simulink library "DQN_Lib"  (R2023b)
settings: Solver=VariableStepAuto  StartTime=0.0  StopTime=10.0  RelTol=1e-3
undefined symbols (not defined in the file): ACDC3, HRM, La, N, R, Ra, sps_AC, SYS, Ts, Ts_dqn, Ts_Power, w, Ws
libraries: DQN_Lib_bak x7
(part 2 of 3)

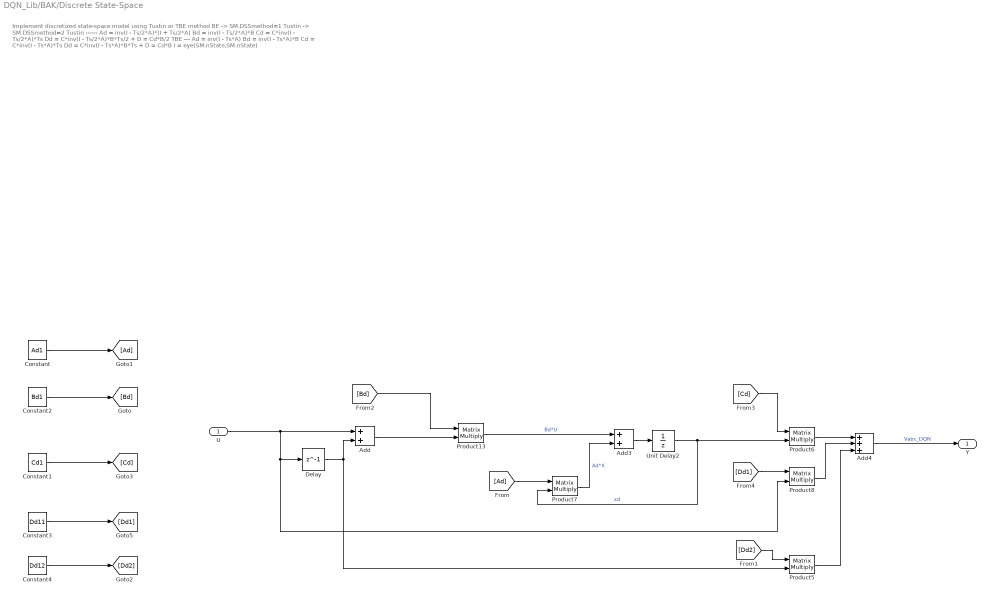
== system DQN_Lib/BAK/Discrete State-Space ==
  note: Implement discretized state-space model using Tustin or TBE method
      |
      | BE      -> SM.DSSmethod=1
      | Tustin  -> SM.DSSmethod=2
      |
      |
      | Tustin
      | ------
      | Ad = inv(I - Ts/2*A)*(I + Ts/2*A)
      | Bd = inv(I - Ts/2*A)*B
      | Cd = C*inv(I - Ts/2*A)*Ts
      | Dd = C*inv(I - Ts/2*A)*B*Ts/2  + D  =  Cd*B/2
      |
      | TBE
      | ---
      | Ad = inv(I - Ts*A)
      | Bd = inv(I - Ts*A)*B
      | Cd = C*inv(I - Ts*A)*Ts
      | Dd = C*inv(I - Ts*A)*B*Ts  + D  =  Cd*B
      |
      | I = eye(SM.nState,SM.nState)
  U : Inport
  Add : Sum
  Add3 : Sum
  Add4 : Sum  Inputs=+++
  Constant : Constant  Value=Ad1
  Constant1 : Constant  Value=Cd1
  Constant2 : Constant  Value=Bd1
  Constant3 : Constant  Value=Dd11
  Constant4 : Constant  Value=Dd12
  Delay : Delay  DelayLength=1  SampleTime=dt
  Product{5..8,13} (5 alike) : Product  Multiplication=Matrix(*)  SaturateOnIntegerOverflow=on  OutDataTypeStr=Inherit: Same as first input
  Unit Delay2 : UnitDelay  InitialCondition=InitVec  SampleTime=dt  HasFrameUpgradeWarning=on
  Y : Outport
  wires:
  Add3/1 -> Unit Delay2/1
  Delay/1 -> Add/2, Product5/2
  [Cd] -> Product6/1
  Unit Delay2/1 -> Product6/2, Product7/2  "xd"
  Product6/1 -> Add4/1
  Add/1 -> Product13/2
  Product7/1 -> Add3/2  "Ad*X"
  Product13/1 -> Add3/1  "Bd*U"
  [Bd] -> Product13/1
  U/1 -> Delay/1, Product8/2, Add/1
  [Dd1] -> Product8/1
  [Ad] -> Product7/1
  Product8/1 -> Add4/2
  Product5/1 -> Add4/3
  [Dd2] -> Product5/1
  Add4/1 -> Y/1  "Vabc_DQN"
  Constant/1 -> [Ad]
  Constant2/1 -> [Bd]
  Constant1/1 -> [Cd]
  Constant3/1 -> [Dd1]
  Constant4/1 -> [Dd2]

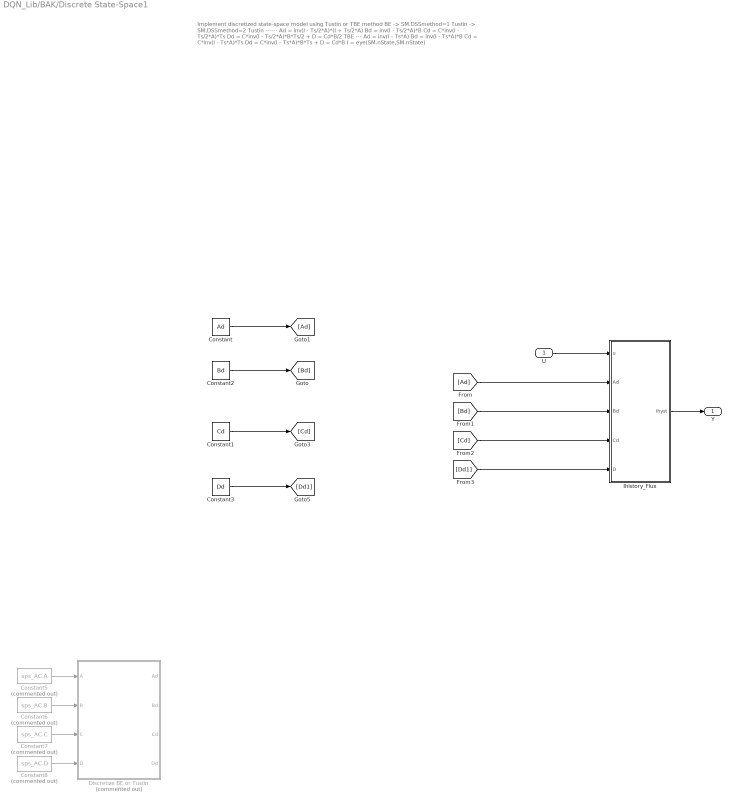
== system DQN_Lib/BAK/Discrete State-Space1 ==
  note: Implement discretized state-space model using Tustin or TBE method
      |
      | BE      -> SM.DSSmethod=1
      | Tustin  -> SM.DSSmethod=2
      |
      |
      | Tustin
      | ------
      | Ad = inv(I - Ts/2*A)*(I + Ts/2*A)
      | Bd = inv(I - Ts/2*A)*B
      | Cd = C*inv(I - Ts/2*A)*Ts
      | Dd = C*inv(I - Ts/2*A)*B*Ts/2  + D  =  Cd*B/2
      |
      | TBE
      | ---
      | Ad = inv(I - Ts*A)
      | Bd = inv(I - Ts*A)*B
      | Cd = C*inv(I - Ts*A)*Ts
      | Dd = C*inv(I - Ts*A)*B*Ts  + D  =  Cd*B
      |
      | I = eye(SM.nState,SM.nState)
  U : Inport
  Constant : Constant  Value=Ad
  Constant1 : Constant  Value=Cd
  Constant2 : Constant  Value=Bd
  Constant3 : Constant  Value=Dd
  Constant5 : Constant  Commented=on  Value=sps_AC.A
  Constant6 : Constant  Commented=on  Value=sps_AC.B
  Constant7 : Constant  Commented=on  Value=sps_AC.C
  Constant8 : Constant  Commented=on  Value=sps_AC.D
  Discretize BE or Tustin : Subsystem  Commented=on  AncestorBlock="DQN_Machines/DQN_Mac_V1/Discretize  BE or Tustin"
  Ihistory_Flux : Subsystem  AncestorBlock=DQN_Machines/DQN_Mac_V1/Ihistory_Flux
  Y : Outport
  wires:
  Constant/1 -> [Ad]
  Constant2/1 -> [Bd]
  Constant1/1 -> [Cd]
  Constant3/1 -> [Dd1]
  Constant7/1 -> Discretize BE or Tustin/3(C)
  Constant6/1 -> Discretize BE or Tustin/2(B)
  Constant8/1 -> Discretize BE or Tustin/4(D)
  Constant5/1 -> Discretize BE or Tustin/1(A)
  U/1 -> Ihistory_Flux/1(u)
  Ihistory_Flux/1(Ihyst) -> Y/1
  [Ad] -> Ihistory_Flux/2(Ad)
  [Bd] -> Ihistory_Flux/3(Bd)
  [Cd] -> Ihistory_Flux/4(Cd)
  [Dd1] -> Ihistory_Flux/5(D)

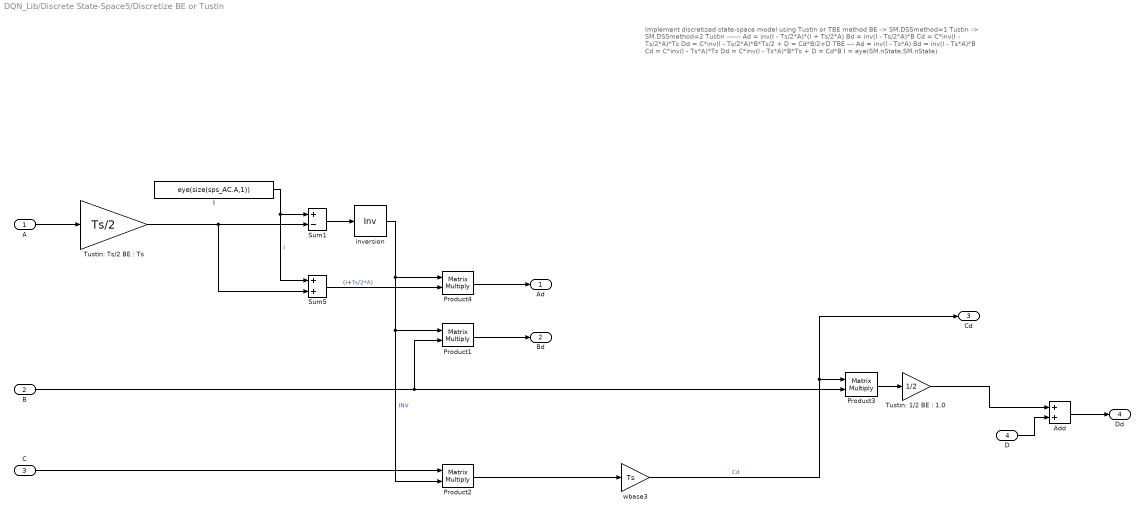
== system DQN_Lib/Discrete State-Space5/Discretize BE or Tustin ==
  note: Implement discretized state-space model using Tustin or TBE method
      |
      | BE      -> SM.DSSmethod=1
      | Tustin  -> SM.DSSmethod=2
      |
      |
      | Tustin
      | ------
      | Ad = inv(I - Ts/2*A)*(I + Ts/2*A)
      | Bd = inv(I - Ts/2*A)*B
      | Cd = C*inv(I - Ts/2*A)*Ts
      | Dd = C*inv(I - Ts/2*A)*B*Ts/2  + D  =  Cd*B/2+D
      |
      | TBE
      | ---
      | Ad = inv(I - Ts*A)
      | Bd = inv(I - Ts*A)*B
      | Cd = C*inv(I - Ts*A)*Ts
      | Dd = C*inv(I - Ts*A)*B*Ts  + D  =  Cd*B
      |
      | I = eye(SM.nState,SM.nState)
  A : Inport
  B : Inport  Port=2
  C : Inport  Port=3
  D : Inport  Port=4
  Add : Sum
  I : Constant  Value=eye(size(sps_AC.A,1))
  Product{1..4} (4 alike) : Product  Multiplication=Matrix(*)  SaturateOnIntegerOverflow=on  OutDataTypeStr=Inherit: Same as first input
  Sum1 : Sum  Inputs=+-  SaturateOnIntegerOverflow=on
  Sum5 : Sum  SaturateOnIntegerOverflow=on
  "Tustin: 1/2 BE : 1.0" : Gain  Gain=1/2  SaturateOnIntegerOverflow=on  OutDataTypeStr=Inherit: Same as input  ParamDataTypeStr=Inherit: Same as input
  "Tustin: Ts/2 BE : Ts" : Gain  Gain=Ts/2  SaturateOnIntegerOverflow=on  OutDataTypeStr=Inherit: Same as input  ParamDataTypeStr=Inherit: Same as input
  inversion : Product  Inputs=/  Multiplication=Matrix(*)  RndMeth=Zero
  wbase3 : Gain  Gain=Ts  SaturateOnIntegerOverflow=on  OutDataTypeStr=Inherit: Same as input  ParamDataTypeStr=Inherit: Same as input
  Ad : Outport  VectorParamsAs1DForOutWhenUnconnected=off
  Bd : Outport  Port=2  VectorParamsAs1DForOutWhenUnconnected=off
  Cd : Outport  Port=3  VectorParamsAs1DForOutWhenUnconnected=off
  Dd : Outport  Port=4  VectorParamsAs1DForOutWhenUnconnected=off
  wires:
  D/1 -> Add/2
  Add/1 -> Dd/1
  "Tustin: Ts/2 BE : Ts"/1 -> Sum1/2, Sum5/2
  Product4/1 -> Ad/1
  A/1 -> "Tustin: Ts/2 BE : Ts"/1
  I/1 -> Sum5/1, Sum1/1  "I"
  Sum1/1 -> inversion/1
  inversion/1 -> Product2/2, Product1/1, Product4/1  "INV"
  Sum5/1 -> Product4/2  "(I+Ts/2*A)"
  Product1/1 -> Bd/1
  B/1 -> Product1/2, Product3/2
  C/1 -> Product2/1
  Product3/1 -> "Tustin: 1/2 BE : 1.0"/1
  "Tustin: 1/2 BE : 1.0"/1 -> Add/1
  Product2/1 -> wbase3/1
  wbase3/1 -> Cd/1, Product3/1  "Cd"

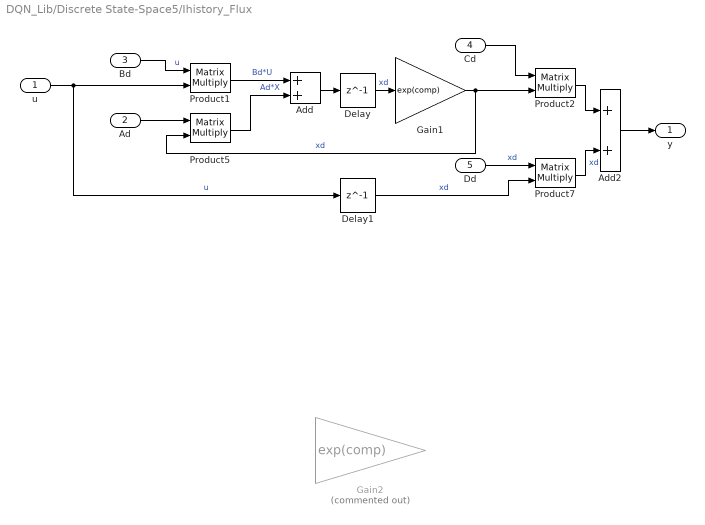
== system DQN_Lib/Discrete State-Space5/Ihistory_Flux ==
  u : Inport
  Ad : Inport  Port=2
  Bd : Inport  Port=3
  Cd : Inport  Port=4
  Dd : Inport  Port=5
  Add : Sum
  Add2 : Sum
  Delay : Delay  DelayLength=1  InitialCondition=InitVec  SampleTime=dt
  Delay1 : Delay  DelayLength=1  InitialCondition=0  SampleTime=dt
  Gain1 : Gain  Gain=exp(comp)
  Gain2 : Gain  Commented=on  Gain=exp(comp)
  Product{1..2,5,7} (4 alike) : Product  Multiplication=Matrix(*)  SaturateOnIntegerOverflow=on  OutDataTypeStr=Inherit: Same as first input
  y : Outport  VectorParamsAs1DForOutWhenUnconnected=off
  wires:
  Dd/1 -> Product7/1  "xd"
  Product7/1 -> Add2/2  "xd"
  Cd/1 -> Product2/1
  Ad/1 -> Product5/1
  Product5/1 -> Add/2  "Ad*X"
  Delay/1 -> Gain1/1  "xd"
  Add/1 -> Delay/1
  Product1/1 -> Add/1  "Bd*U"
  Product2/1 -> Add2/1
  u/1 -> Delay1/1, Product1/2  "u"
  Bd/1 -> Product1/1  "u"
  Add2/1 -> y/1
  Gain1/1 -> Product2/2, Product5/2  "xd"
  Delay1/1 -> Product7/2  "xd"

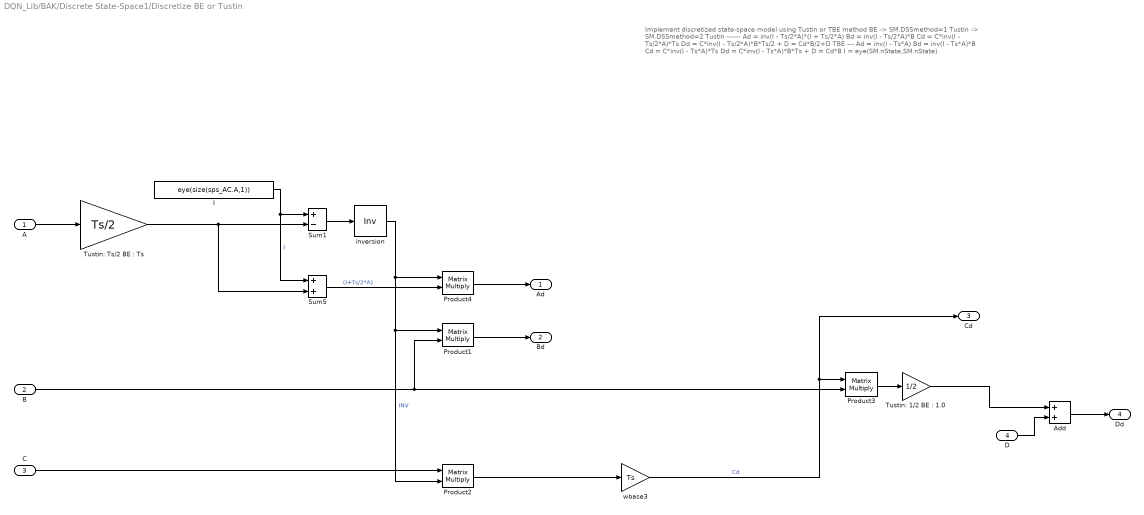
== system DQN_Lib/BAK/Discrete State-Space1/Discretize BE or Tustin ==
  note: Implement discretized state-space model using Tustin or TBE method
      |
      | BE      -> SM.DSSmethod=1
      | Tustin  -> SM.DSSmethod=2
      |
      |
      | Tustin
      | ------
      | Ad = inv(I - Ts/2*A)*(I + Ts/2*A)
      | Bd = inv(I - Ts/2*A)*B
      | Cd = C*inv(I - Ts/2*A)*Ts
      | Dd = C*inv(I - Ts/2*A)*B*Ts/2  + D  =  Cd*B/2+D
      |
      | TBE
      | ---
      | Ad = inv(I - Ts*A)
      | Bd = inv(I - Ts*A)*B
      | Cd = C*inv(I - Ts*A)*Ts
      | Dd = C*inv(I - Ts*A)*B*Ts  + D  =  Cd*B
      |
      | I = eye(SM.nState,SM.nState)
  A : Inport
  B : Inport  Port=2
  C : Inport  Port=3
  D : Inport  Port=4
  Add : Sum
  I : Constant  Value=eye(size(sps_AC.A,1))
  Product{1..4} (4 alike) : Product  Multiplication=Matrix(*)  SaturateOnIntegerOverflow=on  OutDataTypeStr=Inherit: Same as first input
  Sum1 : Sum  Inputs=+-  SaturateOnIntegerOverflow=on
  Sum5 : Sum  SaturateOnIntegerOverflow=on
  "Tustin: 1/2 BE : 1.0" : Gain  Gain=1/2  SaturateOnIntegerOverflow=on  OutDataTypeStr=Inherit: Same as input  ParamDataTypeStr=Inherit: Same as input
  "Tustin: Ts/2 BE : Ts" : Gain  Gain=Ts/2  SaturateOnIntegerOverflow=on  OutDataTypeStr=Inherit: Same as input  ParamDataTypeStr=Inherit: Same as input
  inversion : Product  Inputs=/  Multiplication=Matrix(*)  RndMeth=Zero
  wbase3 : Gain  Gain=Ts  SaturateOnIntegerOverflow=on  OutDataTypeStr=Inherit: Same as input  ParamDataTypeStr=Inherit: Same as input
  Ad : Outport  VectorParamsAs1DForOutWhenUnconnected=off
  Bd : Outport  Port=2  VectorParamsAs1DForOutWhenUnconnected=off
  Cd : Outport  Port=3  VectorParamsAs1DForOutWhenUnconnected=off
  Dd : Outport  Port=4  VectorParamsAs1DForOutWhenUnconnected=off
  wires:
  wbase3/1 -> Product3/1, Cd/1  "Cd"
  Product2/1 -> wbase3/1
  "Tustin: 1/2 BE : 1.0"/1 -> Add/1
  Product3/1 -> "Tustin: 1/2 BE : 1.0"/1
  C/1 -> Product2/1
  B/1 -> Product3/2, Product1/2
  Product1/1 -> Bd/1
  Sum5/1 -> Product4/2  "(I+Ts/2*A)"
  inversion/1 -> Product4/1, Product1/1, Product2/2  "INV"
  Sum1/1 -> inversion/1
  I/1 -> Sum1/1, Sum5/1  "I"
  A/1 -> "Tustin: Ts/2 BE : Ts"/1
  Product4/1 -> Ad/1
  "Tustin: Ts/2 BE : Ts"/1 -> Sum5/2, Sum1/2
  Add/1 -> Dd/1
  D/1 -> Add/2

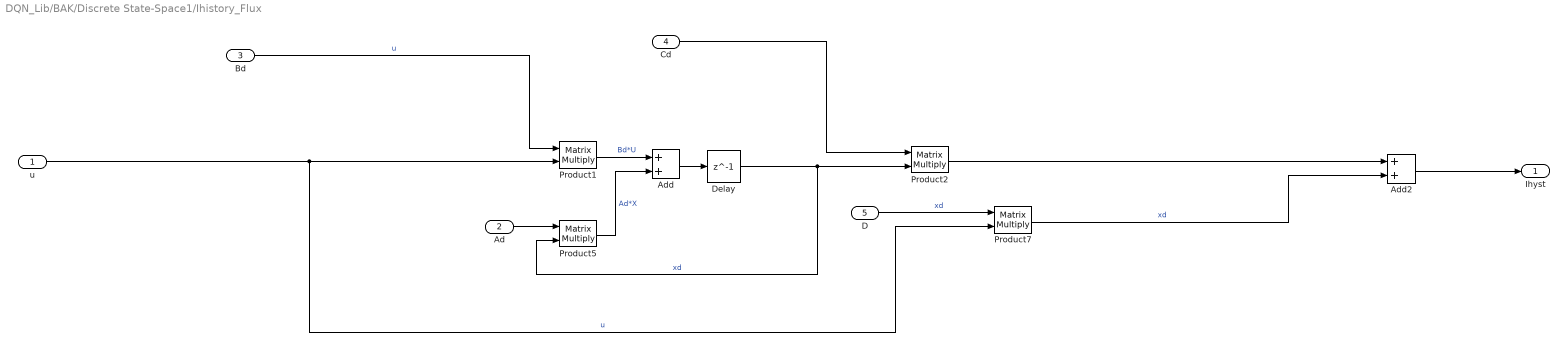
== system DQN_Lib/BAK/Discrete State-Space1/Ihistory_Flux ==
  u : Inport
  Ad : Inport  Port=2
  Bd : Inport  Port=3
  Cd : Inport  Port=4
  D : Inport  Port=5
  Add : Sum
  Add2 : Sum
  Delay : Delay  DelayLength=1  InitialCondition=InitVec  SampleTime=dt
  Product{1..2,5,7} (4 alike) : Product  Multiplication=Matrix(*)  SaturateOnIntegerOverflow=on  OutDataTypeStr=Inherit: Same as first input
  Ihyst : Outport  VectorParamsAs1DForOutWhenUnconnected=off
  wires:
  Add2/1 -> Ihyst/1
  Bd/1 -> Product1/1  "u"
  u/1 -> Product7/2, Product1/2  "u"
  Product2/1 -> Add2/1
  Product1/1 -> Add/1  "Bd*U"
  Add/1 -> Delay/1
  Delay/1 -> Product2/2, Product5/2  "xd"
  Product5/1 -> Add/2  "Ad*X"
  Ad/1 -> Product5/1
  Cd/1 -> Product2/1
  Product7/1 -> Add2/2  "xd"
  D/1 -> Product7/1  "xd"

== matlab function DQN_Lib/MATLAB Function2 ==
  data: Ydcpnz_c output; X_DQN input; N parameter
function Ydcpnz_c  = fDQN012C(X_DQN, N)
        
            if(size(X_DQN,2) < 1)
                error('Wrong size!');
            end
            
            % N = size(X_DQN,1);
            % 
            % if(size(X_DQN,1) == 6 && size(X_DQN,2) == 1)
            %     N = 1;
            %     X_DQN = X_DQN';
            % end
        
            Ydcpnz_c = complex(zeros(3,N+1));
        
            for i = 1 : N+1
             
                if(i>1)
                    Ydcpnz_c(1,i) = (X_DQN(i,1)) + 1i*X_DQN(i,4);
                    Ydcpnz_c(2,i) = (-X_DQN(i,2)) + 1i*X_DQN(i,5);
                    Ydcpnz_c(3,i) = (X_DQN(i,3)) + 1i*X_DQN(i,6);
                else
        
                    Ydcpnz_c(1,i) = 0.5*(X_DQN(i,4) - 1i*X_DQN(i,1));
                    Ydcpnz_c(2,i) = 0.5*(X_DQN(i,5) + 1i*X_DQN(i,2));
                    Ydcpnz_c(3,i) =     (X_DQN(i,6) + 1i*X_DQN(i,3));
                end
            
            end
        
        
        end

== matlab function DQN_Lib/Subsystem1/DQN Mux ==
  data: u input; y output; N parameter
function y = MUX_vec(u, N)

    y = zeros((N+1)*6,1);

    for i = 1 : (N+1)*6


        if(i <= 1*(N+1)) %dp
            y(i) = u(mod(i+N,N+1)*6+1);
        elseif(i > 1*(N+1) && i <= 2*(N+1))
            y(i) = u(mod(i+N,N+1)*6+2);
        elseif(i > 2*(N+1) && i <= 3*(N+1))
            y(i) = u(mod(i+N,N+1)*6+3);
        elseif(i > 3*(N+1) && i <= 4*(N+1))
            y(i) = u(mod(i+N,N+1)*6+4);
        elseif(i > 4*(N+1) && i <= 5*(N+1))
            y(i) = u(mod(i+N,N+1)*6+5);
        elseif(i > 5*(N+1) && i <= 6*(N+1))
            y(i) = u(mod(i+N,N+1)*6+6);
        end
    end
    
end

== matlab function DQN_Lib/ABC2PNZ ==
  data: Xabc input; Ypnz output
function Ypnz  = ABC2PNZ(Xabc)
    persistent Sas;

    if(isempty(Sas)) 
        a = -0.5+0.866i;
        a2 = -0.5-0.866i;
        Sas = [1,a,a2;1,a2,a;1,1,1]/3;
    end
    
    Ypnz = Sas*Xabc/Sas;

end

== matlab function DQN_Lib/Int_DQN_fdbk/Int_d_2N_2 ==
  settings: updateMethod=DISCRETE
  data: Zdp output; Xdp input; Xdn input; Xdz input; Xqp input; Xqn input; Xqz input; Zdn output; N parameter; dt parameter; w parameter; Zdz output; Zqp output; Zqn output; Zqz output; R parameter; iL parameter; SW parameter
function [Zdp,Zdn,Zdz,Zqp,Zqn,Zqz]  = IntDQN(Xdp, Xdn, Xdz, Xqp, Xqn, Xqz, N, dt, w, R, iL, SW)

    persistent Zdc_old;    
    persistent Xdc_old;   
    persistent Zdp_old;    
    persistent Zqp_old;    
    persistent Zdn_old;    
    persistent Zqn_old;    
    persistent Zdz_old;    
    persistent Zqz_old;  
    persistent Krl1;
    persistent Krl2;
       
    persistent dt2;
    persistent range;
       
    Xdc = zeros(6,1);
    Zdc = zeros(6,1);
    
    Xdc(1) = Xdp(1);
    Xdc(2) = Xdn(1);
    Xdc(3) = Xdz(1);
    Xdc(4) = Xqp(1);
    Xdc(5) = Xqn(1);
    Xdc(6) = Xqz(1);

    Xdp = [Xdp(2:end); zeros(N-numel(Xdp)+1,1)];
    Xqp = [Xqp(2:end); zeros(N-numel(Xqp)+1,1)];
    Xdn = [Xdn(2:end); zeros(N-numel(Xdn)+1,1)];
    Xqn = [Xqn(2:end); zeros(N-numel(Xqn)+1,1)];
    Xdz = [Xdz(2:end); zeros(N-numel(Xdz)+1,1)];
    Xqz = [Xqz(2:end); zeros(N-numel(Xqz)+1,1)];
       
    Zdp = zeros(N+1,1);
    Zdn = zeros(N+1,1);
    Zqp = zeros(N+1,1);
    Zqn = zeros(N+1,1);
    Zdz = zeros(N+1,1);
    Zqz = zeros(N+1,1);
       
    if(isempty(Zdp_old)) 
        Zdc_old  = zeros(6,1); %Zdc_old  = InitInt';
        Xdc_old  = zeros(6,1);
        
        Zdp_old  = zeros(N,1);% Zdp_old(1) = InitInt(1);
        Zdn_old  = zeros(N,1);% Zdn_old(1) = InitInt(2);
        Zdz_old  = zeros(N,1);% Zdz_old(1) = InitInt(3);
        Zqp_old  = zeros(N,1);% Zqp_old(1) = InitInt(4);
        Zqn_old  = zeros(N,1);% Zqn_old(1) = InitInt(5);
        Zqz_old  = zeros(N,1);% Zqz_old(1) = InitInt(6);
        
        dt2 = dt/2;  
        range = N; 
        
        if(SW)
            Krl1 = (iL/(1+dt2*R*iL));
            Krl2 = (1-dt2*R*iL)/(1+dt2*R*iL);
        else
            Krl1 = 1;
            Krl2 = 1;
        end
        
    end

    
    
    %Zdc(:) = dt2*(Xdc(:)+Xdc_old(:))+Zdc_old(:);
    Zdc(:) = Krl1*dt2*(Xdc(:)+Xdc_old(:))+Krl2*Zdc_old(:);
    
    
    Zdc_old = Zdc;
    Xdc_old = Xdc;
    
    if(N>0)
              
        for i = 1 : range

            wn =  i * w;
            wndt2 = wn*dt2;
            A = 2*dt2/(1+wndt2^2);
            B = (1-wndt2^2)/(1+wndt2^2);

            %%% NEG %%%
            Zdp(i) = Krl1*A*(Xdp(i)+wndt2*Xqp(i))+Krl2*(B*Zdp_old(i)+A*wn*Zqp_old(i));
            Zqp(i) = Krl1*A*(Xqp(i)-wndt2*Xdp(i))+Krl2*(B*Zqp_old(i)-A*wn*Zdp_old(i));

            Zdp_old(i) = Zdp(i);
            Zqp_old(i) = Zqp(i); 


            %%% NEG %%%
            Zdn(i) = Krl1*A*(Xdn(i)-wndt2*Xqn(i))+Krl2*(B*Zdn_old(i)-A*wn*Zqn_old(i));
            Zqn(i) = Krl1*A*(Xqn(i)+wndt2*Xdn(i))+Krl2*(B*Zqn_old(i)+A*wn*Zdn_old(i));

            Zdn_old(i) = Zdn(i);
            Zqn_old(i) = Zqn(i); 

            %%% ZERO %%%
            Zdz(i) = Krl1*A*(Xdz(i)+wndt2*Xqz(i))+Krl2*(B*Zdz_old(i)+A*wn*Zqz_old(i));
            Zqz(i) = Krl1*A*(Xqz(i)-wndt2*Xdz(i))+Krl2*(B*Zqz_old(i)-A*wn*Zdz_old(i));

            Zdz_old(i) = Zdz(i);
            Zqz_old(i) = Zqz(i); 
        end

        Zdp(2:end) = Zdp(1:end-1);
        Zdn(2:end) = Zdn(1:end-1);
        Zdz(2:end) = Zdz(1:end-1);
        Zqp(2:end) = Zqp(1:end-1);
        Zqn(2:end) = Zqn(1:end-1);
        Zqz(2:end) = Zqz(1:end-1);


    end
    
    Zdp(1)     = Zdc(1);
    Zdn(1)     = Zdc(2);
    Zdz(1)     = Zdc(3);
    Zqp(1)     = Zdc(4);
    Zqn(1)     = Zdc(5);
    Zqz(1)     = Zdc(6);
end

== matlab function DQN_Lib/MATLAB Function4 ==
  data: Xdcpnz_c input; Y_DQN output
function Y_DQN  = f012C2DQN(Xdcpnz_c)

    if(size(Xdcpnz_c,2) < 2)
        error('Wrong size!');
    end
    
    N = size(Xdcpnz_c,2)-1;
    Y_DQN = zeros(N+1,6);

    Y_DQN(1,4) =  2*real(Xdcpnz_c(1,1));
    Y_DQN(1,5) =  2*real(Xdcpnz_c(2,1));
    Y_DQN(1,6) =  real(Xdcpnz_c(3,1));

    Y_DQN(1,1) =  -2*imag(Xdcpnz_c(1,1));
    Y_DQN(1,2) =  2*imag(Xdcpnz_c(2,1));
    Y_DQN(1,3) =  imag(Xdcpnz_c(3,1));
    
    for i = 2 : N + 1
    
        Y_DQN(i,1) =  real(Xdcpnz_c(1,i));
        Y_DQN(i,2) = -real(Xdcpnz_c(2,i));
        Y_DQN(i,3) =  real(Xdcpnz_c(3,i));

        Y_DQN(i,4) =  imag(Xdcpnz_c(1,i));
        Y_DQN(i,5) =  imag(Xdcpnz_c(2,i));
        Y_DQN(i,6) =  imag(Xdcpnz_c(3,i));
    
    end


end

== matlab function DQN_Lib/Mult_DQNc_Mat ==
  data: Xdcpnz_c input; Ydcpnz_c input; N parameter; HrmDbl parameter; Zdcpnz_c output
function Zdcpnz_c    = fMultDQNc(Xdcpnz_c, Ydcpnz_c, N, HrmDbl)
    Zdcpnz_c = complex(zeros(3,2*N+1));

    persistent T132;
    persistent T213;
    persistent T231;
    persistent T321;
    persistent T312;
    persistent Sas;
    persistent Ssa;

    if(isempty(T132)) 
        T132 = [1 0 0; 0 0 1; 0 1 0];
        T213 = [0 1 0; 1 0 0; 0 0 1];
        T231 = [0 1 0; 0 0 1; 1 0 0];
        T321 = [0 0 1; 0 1 0; 1 0 0];
        T312 = [0 0 1; 1 0 0; 0 1 0];

        a = -0.5+0.866i;
        a2 = -0.5-0.866i;
        Sas = [1,a,a2;1,a2,a;1,1,1]/3;
        Ssa = eye(3)/(Sas);
    end

%%%%%%%%%%%%%%%%%%%%%%%%%%%%%%

    Zdcpnz_c(:,1) = Sas*(Ssa*Xdcpnz_c(:,1).*Ssa*Ydcpnz_c(:,1));

    sX = size(Xdcpnz_c,2);
    Xdcpnz_c = [Xdcpnz_c zeros(3,N+1-sX)];

    sY = size(Ydcpnz_c,2);
    Ydcpnz_c = [Ydcpnz_c zeros(3,N+1-sY)];

       
    for h = 1 : 2*N
        if(h<=N)

            Zdcpnz_c(3,1) = Zdcpnz_c(3,1) + 0.5*real(Xdcpnz_c(:,h+1)'*Ydcpnz_c(:,h+1));


            Zdcpnz_c(3,2*h+1) = Zdcpnz_c(3,2*h+1) + 0.5*Xdcpnz_c(1,h+1)*Ydcpnz_c(2,h+1)*exp(-1i*pi/2);

            Zdcpnz_c(1:2,1) = Zdcpnz_c(1:2,1) + 0.25*abs(Xdcpnz_c(1,h+1))*abs(Ydcpnz_c(2,h+1))*[1;1].*exp(1i*((-angle(Xdcpnz_c(1,h+1))+angle(Ydcpnz_c(2,h+1)))*[1;-1]));
            Zdcpnz_c(1:2,1) = Zdcpnz_c(1:2,1) + 0.25*abs(Xdcpnz_c(1,h+1))*abs(Ydcpnz_c(3,h+1))*[1;1].*exp(1i*((-angle(Xdcpnz_c(1,h+1))+angle(Ydcpnz_c(3,h+1)))*[-1;1]));


            Zdcpnz_c(3,2*h+1) = Zdcpnz_c(3,2*h+1) + 0.5*Xdcpnz_c(2,h+1)*Ydcpnz_c(1,h+1)*exp(-1i*pi/2);


            Zdcpnz_c(1:2,1) = Zdcpnz_c(1:2,1) + 0.25*abs(Xdcpnz_c(2,h+1))*abs(Ydcpnz_c(1,h+1))*[1;1].*exp(1i*((-angle(Xdcpnz_c(2,h+1))+angle(Ydcpnz_c(1,h+1)))*[-1;1]));
            Zdcpnz_c(1:2,1) = Zdcpnz_c(1:2,1) + 0.25*abs(Xdcpnz_c(2,h+1))*abs(Ydcpnz_c(3,h+1))*[1;1].*exp(1i*((-angle(Xdcpnz_c(2,h+1))+angle(Ydcpnz_c(3,h+1)))*[1;-1]));
            
            Zdcpnz_c(1:2,1) = Zdcpnz_c(1:2,1) + 0.25*abs(Xdcpnz_c(3,h+1))*abs(Ydcpnz_c(1,h+1))*[1;1].*exp(1i*((-angle(Xdcpnz_c(3,h+1))+angle(Ydcpnz_c(1,h+1)))*[1;-1]));
            Zdcpnz_c(1:2,1) = Zdcpnz_c(1:2,1) + 0.25*abs(Xdcpnz_c(3,h+1))*abs(Ydcpnz_c(2,h+1))*[1;1].*exp(1i*((-angle(Xdcpnz_c(3,h+1))+angle(Ydcpnz_c(2,h+1)))*[-1;+1]));

            %%%%%%%%%%%%%%%%% POSITIVE (Ydc*Xp) %%%%%%%%%%%%%%%%%%%
            Zdcpnz_c(:,h+1) = Zdcpnz_c(:,h+1) + T312*Ydcpnz_c(:,1)*Xdcpnz_c(1,h+1); %[0 0 1; 1 0 0; 0 1 0]
            %%%%%%%%%%%%%%%%% POSITIVE (Xdc*Yp) %%%%%%%%%%%%%%%%%%%
            Zdcpnz_c(:,h+1) = Zdcpnz_c(:,h+1) + T312*Xdcpnz_c(:,1)*Ydcpnz_c(1,h+1);
            %%%%%%%%%%%%%%%%% NEGATIVE (Ydc*Xn) %%%%%%%%%%%%%%%%%%%
            Zdcpnz_c(:,h+1) = Zdcpnz_c(:,h+1) + T231*Ydcpnz_c(:,1)*Xdcpnz_c(2,h+1);
            %%%%%%%%%%%%%%%%% NEGATIVE (Xdc*Yn) %%%%%%%%%%%%%%%%%%%
            Zdcpnz_c(:,h+1) = Zdcpnz_c(:,h+1) + T231*Xdcpnz_c(:,1)*Ydcpnz_c(2,h+1);
            %%%%%%%%%%%%%%%%%%%%%%%%%%%%%%%%%%%%%%%%%%%%%%%%%%%%%%
            Zdcpnz_c(:,h+1) = Zdcpnz_c(:,h+1) + Ydcpnz_c(:,1)*Xdcpnz_c(3,h+1);
            %%%%%%%%%%%%%%%%%%%%%%%%%%%%%%%%%%%%%%%%%%%%%%%%%%%%%%
            Zdcpnz_c(:,h+1) = Zdcpnz_c(:,h+1) + Xdcpnz_c(:,1)*Ydcpnz_c(3,h+1);
            
%%%%%%%%%%%%%%%%%%%%%% h<=N ODD %%%%%%%%%%%%%%%%%%%%%%%%%%%%%%%%%%%%%%%%%
            if(mod(h,2)==1) 
                %%%%%%%%%%%%%%%%% D3p (3ph+) %%%%%%%%%%%%%%%%%%%%%%%

                %&%%%%%%%%%%%%%%%%%%%%%%%%%% PP + NN %%%%%%%%%%%%%%%%%%%%%%%%%%%
                for i = 1 : h - 1
                   Zdcpnz_c(1,h+1) = Zdcpnz_c(1,h+1) +    0.5*( real(Xdcpnz_c(2,i+1))*imag(Ydcpnz_c(2,h-i+1)) + imag(Xdcpnz_c(2,i+1))*real(Ydcpnz_c(2,h-i+1)) );
                   Zdcpnz_c(1,h+1) = Zdcpnz_c(1,h+1) + 1i*0.5*( -real(Xdcpnz_c(2,i+1))*real(Ydcpnz_c(2,h-i+1)) + imag(Xdcpnz_c(2,i+1))*imag(Ydcpnz_c(2,h-i+1)) );

                   Zdcpnz_c(2,h+1) = Zdcpnz_c(2,h+1) +    0.5*( real(Xdcpnz_c(1,i+1))*imag(Ydcpnz_c(1,h-i+1)) + imag(Xdcpnz_c(1,i+1))*real(Ydcpnz_c(1,h-i+1)) );
                   Zdcpnz_c(2,h+1) = Zdcpnz_c(2,h+1) + 1i*0.5*( -real(Xdcpnz_c(1,i+1))*real(Ydcpnz_c(1,h-i+1)) + imag(Xdcpnz_c(1,i+1))*imag(Ydcpnz_c(1,h-i+1)) );
                end

                for i = 1 : N - h

                    Zdcpnz_c(3,h+1) = Zdcpnz_c(3,h+1) -    imag(0.5*Xdcpnz_c(1:2,i+1)'*Ydcpnz_c(1:2,i+h+1)) -    imag(0.5*Ydcpnz_c(1:2,i+1)'*Xdcpnz_c(1:2,i+h+1));
                    Zdcpnz_c(3,h+1) = Zdcpnz_c(3,h+1) + 1i*real(0.5*Xdcpnz_c(1:2,i+1)'*Ydcpnz_c(1:2,i+h+1)) + 1i*real(0.5*Ydcpnz_c(1:2,i+1)'*Xdcpnz_c(1:2,i+h+1));

                end
                %&%%%%%%%%%%%%%%%%%%%%%%%%%% PP + NN %%%%%%%%%%%%%%%%%%%%%%%%%%%

                for k = 1 : (N + mod(N+1,2) - h)/2
                    i = 2*k-1;
                    j = i+h;

                    Zdcpnz_c(1,h+1) = Zdcpnz_c(1,h+1) + (0.5*(Xdcpnz_c(:,i+1)'*T132*T213*Ydcpnz_c(:,j+1))*exp(+1i*pi/2)) ...
                                                      + (0.5*(Xdcpnz_c(:,j+1)'*T213*T132*Ydcpnz_c(:,i+1))*exp(-1i*pi/2))';

                    Zdcpnz_c(2,h+1) = Zdcpnz_c(2,h+1) + (0.5*(Xdcpnz_c(:,i+1)'*T132*T321*Ydcpnz_c(:,j+1))*exp(+1i*pi/2)) ...
                                                      + (0.5*(Xdcpnz_c(:,j+1)'*T321*T132*Ydcpnz_c(:,i+1))*exp(-1i*pi/2))';

                    Zdcpnz_c(3,h+1) = Zdcpnz_c(3,h+1) + (0.5*Xdcpnz_c(3,i+1)'*Ydcpnz_c(3,j+1)*exp(1i*pi/2)) ...
                                                      - (0.5*Xdcpnz_c(3,j+1)'*Ydcpnz_c(3,i+1)*exp(1i*pi/2))';
                end

                for k = 1 : (N + mod(N,2) - h - 1)/2
                    i = 2*k;
                    j = i+h;
                    
                    Zdcpnz_c(1,h+1) = Zdcpnz_c(1,h+1) + (0.5*(Xdcpnz_c(:,i+1)'*T132*T213*Ydcpnz_c(:,j+1))*exp(+1i*pi/2)) ...
                                                      + (0.5*(Xdcpnz_c(:,j+1)'*T213*T132*Ydcpnz_c(:,i+1))*exp(-1i*pi/2))';

                    Zdcpnz_c(2,h+1) = Zdcpnz_c(2,h+1) + (0.5*(Xdcpnz_c(:,i+1)'*T132*T321*Ydcpnz_c(:,j+1))*exp(+1i*pi/2)) ...
                                                      + (0.5*(Xdcpnz_c(:,j+1)'*T321*T132*Ydcpnz_c(:,i+1))*exp(-1i*pi/2))';

                    Zdcpnz_c(3,h+1) = Zdcpnz_c(3,h+1) + (0.5*Xdcpnz_c(3,i+1)'*Ydcpnz_c(3,j+1)*exp(1i*pi/2)) ...
                                                      - (0.5*Xdcpnz_c(3,j+1)'*Ydcpnz_c(3,i+1)*exp(1i*pi/2))';
                end

                for k = (h-1)/2:-1:1
                    i = k;
                    j = h-i;  

                    Zdcpnz_c(3,h+1) = Zdcpnz_c(3,h+1) + 0.5*(real(Xdcpnz_c(:,i+1))'*T213*imag(Ydcpnz_c(:,j+1)) + imag(Xdcpnz_c(:,i+1))'*T213*real(Ydcpnz_c(:,j+1)) ...
                                                           + real(Xdcpnz_c(:,j+1))'*T213*imag(Ydcpnz_c(:,i+1)) + imag(Xdcpnz_c(:,j+1))'*T213*real(Ydcpnz_c(:,i+1)));
                                                                                       
                    Zdcpnz_c(3,h+1) = Zdcpnz_c(3,h+1) + 1i*0.5*(-real(Xdcpnz_c(:,i+1))'*T213*real(Ydcpnz_c(:,j+1)) + imag(Xdcpnz_c(:,i+1))'*T213*imag(Ydcpnz_c(:,j+1)) ...
                                                           - real(Xdcpnz_c(:,j+1))'*T213*real(Ydcpnz_c(:,i+1)) + imag(Xdcpnz_c(:,j+1))'*T213*imag(Ydcpnz_c(:,i+1)));

                    Zdcpnz_c(1,h+1) = Zdcpnz_c(1,h+1) + 0.5*(real(Xdcpnz_c([1,3],i+1))'*[0 1; 1 0]*imag(Ydcpnz_c([1,3],j+1)) + imag(Xdcpnz_c([1,3],i+1))'*[0 1; 1 0]*real(Ydcpnz_c([1,3],j+1)) ...
                                                           + real(Xdcpnz_c([1,3],j+1))'*[0 1; 1 0]*imag(Ydcpnz_c([1,3],i+1)) + imag(Xdcpnz_c([1,3],j+1))'*[0 1; 1 0]*real(Ydcpnz_c([1,3],i+1)) );

                    Zdcpnz_c(1,h+1) = Zdcpnz_c(1,h+1) + 1i*0.5*(-real(Xdcpnz_c([1,3],i+1))'*[0 1; 1 0]*real(Ydcpnz_c([1,3],j+1)) + imag(Xdcpnz_c([1,3],i+1))'*[0 1; 1 0]*imag(Ydcpnz_c([1,3],j+1)) ...
                                                              - real(Xdcpnz_c([1,3],j+1))'*[0 1; 1 0]*real(Ydcpnz_c([1,3],i+1)) + imag(Xdcpnz_c([1,3],j+1))'*[0 1; 1 0]*imag(Ydcpnz_c([1,3],i+1)) );

                    Zdcpnz_c(2,h+1) = Zdcpnz_c(2,h+1) + 0.5*(real(Xdcpnz_c([2,3],i+1))'*[0 1; 1 0]*imag(Ydcpnz_c([2,3],j+1)) + imag(Xdcpnz_c([2,3],i+1))'*[0 1; 1 0]*real(Ydcpnz_c([2,3],j+1)) ...
                                                           + real(Xdcpnz_c([2,3],j+1))'*[0 1; 1 0]*imag(Ydcpnz_c([2,3],i+1)) + imag(Xdcpnz_c([2,3],j+1))'*[0 1; 1 0]*real(Ydcpnz_c([2,3],i+1)) );

                    Zdcpnz_c(2,h+1) = Zdcpnz_c(2,h+1) + 1i*0.5*(-real(Xdcpnz_c([2,3],i+1))'*[0 1; 1 0]*real(Ydcpnz_c([2,3],j+1)) + imag(Xdcpnz_c([2,3],i+1))'*[0 1; 1 0]*imag(Ydcpnz_c([2,3],j+1)) ...
                                                              - real(Xdcpnz_c([2,3],j+1))'*[0 1; 1 0]*real(Ydcpnz_c([2,3],i+1)) + imag(Xdcpnz_c([2,3],j+1))'*[0 1; 1 0]*imag(Ydcpnz_c([2,3],i+1)) );

                end
%%%%%%%%%%%%%%%%%%%%%% h<=N EVEN %%%%%%%%%%%%%%%%%%%%%%%%%%%%%%%%%%%%%%%%%           
            else  

                Zdcpnz_c(3,h+1) = Zdcpnz_c(3,h+1) + 0.5*imag(Xdcpnz_c(3,h/2+1)*Ydcpnz_c(3,h/2+1))           -0.5*1i*real(Xdcpnz_c(3,h/2+1)*Ydcpnz_c(3,h/2+1));
                Zdcpnz_c(1,h+1) = Zdcpnz_c(1,h+1) + 0.5*real(Xdcpnz_c(:,h/2+1))'*T321*imag(Ydcpnz_c(:,h/2+1)) + 0.5*imag(Xdcpnz_c(:,h/2+1))'*T321*real(Ydcpnz_c(:,h/2+1));
                Zdcpnz_c(1,h+1) = Zdcpnz_c(1,h+1) - 0.5*1i*real(Xdcpnz_c(:,h/2+1))'*T321*real(Ydcpnz_c(:,h/2+1)) + 0.5*1i*imag(Xdcpnz_c(:,h/2+1))'*T321*imag(Ydcpnz_c(:,h/2+1));
                Zdcpnz_c(2,h+1) = Zdcpnz_c(2,h+1) + 0.5*real(Xdcpnz_c(:,h/2+1))'*T132*imag(Ydcpnz_c(:,h/2+1)) + 0.5*imag(Xdcpnz_c(:,h/2+1))'*T132*real(Ydcpnz_c(:,h/2+1));
                Zdcpnz_c(2,h+1) = Zdcpnz_c(2,h+1) - 0.5*1i*real(Xdcpnz_c(:,h/2+1))'*T132*real(Ydcpnz_c(:,h/2+1)) + 0.5*1i*imag(Xdcpnz_c(:,h/2+1))'*T132*imag(Ydcpnz_c(:,h/2+1));
                
                for k = 1:N-h
                    i = k;
                    j = h+i;

                    Zdcpnz_c(1,h+1) = Zdcpnz_c(1,h+1) + 0.5*( - real(Xdcpnz_c(:,i+1))'*T231*imag(Ydcpnz_c(:,j+1)) + imag(Xdcpnz_c(:,i+1))'*T231*real(Ydcpnz_c(:,j+1)) ...
                                                              + real(Xdcpnz_c(:,j+1))'*T312*imag(Ydcpnz_c(:,i+1)) - imag(Xdcpnz_c(:,j+1))'*T312*real(Ydcpnz_c(:,i+1)));

                    Zdcpnz_c(1,h+1) = Zdcpnz_c(1,h+1) + 0.5*1i*( + real(Xdcpnz_c(:,i+1))'*T231*real(Ydcpnz_c(:,j+1)) + imag(Xdcpnz_c(:,i+1))'*T231*imag(Ydcpnz_c(:,j+1)) ...
                                                                 + real(Xdcpnz_c(:,j+1))'*T312*real(Ydcpnz_c(:,i+1)) + imag(Xdcpnz_c(:,j+1))'*T312*imag(Ydcpnz_c(:,i+1)));

                    Zdcpnz_c(2,h+1) = Zdcpnz_c(2,h+1) + 0.5*( - real(Xdcpnz_c(:,i+1))'*T312*imag(Ydcpnz_c(:,j+1)) + imag(Xdcpnz_c(:,i+1))'*T312*real(Ydcpnz_c(:,j+1)) ...
                                                              + real(Xdcpnz_c(:,j+1))'*T231*imag(Ydcpnz_c(:,i+1)) - imag(Xdcpnz_c(:,j+1))'*T231*real(Ydcpnz_c(:,i+1)));

                    Zdcpnz_c(2,h+1) = Zdcpnz_c(2,h+1) + 1i*0.5*( + real(Xdcpnz_c(:,i+1))'*T312*real(Ydcpnz_c(:,j+1)) + imag(Xdcpnz_c(:,i+1))'*T312*imag(Ydcpnz_c(:,j+1)) ...
                                                              + real(Xdcpnz_c(:,j+1))'*T231*real(Ydcpnz_c(:,i+1)) + imag(Xdcpnz_c(:,j+1))'*T231*imag(Ydcpnz_c(:,i+1)));

                    Zdcpnz_c(3,h+1) = Zdcpnz_c(3,h+1) + 0.5*(-real(Xdcpnz_c(:,i+1))'*imag(Ydcpnz_c(:,j+1))+imag(Xdcpnz_c(:,i+1))'*real(Ydcpnz_c(:,j+1)) ...
                                                             +real(Xdcpnz_c(:,j+1))'*imag(Ydcpnz_c(:,i+1))-imag(Xdcpnz_c(:,j+1))'*real(Ydcpnz_c(:,i+1)));

                    Zdcpnz_c(3,h+1) = Zdcpnz_c(3,h+1) + 0.5*1i*(+real(Xdcpnz_c(:,i+1))'*real(Ydcpnz_c(:,j+1))+imag(Xdcpnz_c(:,i+1))'*imag(Ydcpnz_c(:,j+1)) ...
                                                             +real(Xdcpnz_c(:,j+1))'*real(Ydcpnz_c(:,i+1))+imag(Xdcpnz_c(:,j+1))'*imag(Ydcpnz_c(:,i+1)));

                end

                for k = h/2-1:-1:1
                    i = k;
                    j = h-i;   

                    Zdcpnz_c(3,h+1) = Zdcpnz_c(3,h+1) +    0.5*(+real(Xdcpnz_c(:,i+1))'*T213*imag(Ydcpnz_c(:,j+1)) + real(Xdcpnz_c(:,j+1))'*T213*imag(Ydcpnz_c(:,i+1)) + imag(Xdcpnz_c(:,i+1))'*T213*real(Ydcpnz_c(:,j+1)) + imag(Xdcpnz_c(:,j+1))'*T213*real(Ydcpnz_c(:,i+1)));

                    Zdcpnz_c(3,h+1) = Zdcpnz_c(3,h+1) + 1i*0.5*(-real(Xdcpnz_c(:,i+1))'*T213*real(Ydcpnz_c(:,j+1)) - real(Xdcpnz_c(:,j+1))'*T213*real(Ydcpnz_c(:,i+1)) + imag(Xdcpnz_c(:,i+1))'*T213*imag(Ydcpnz_c(:,j+1)) + imag(Xdcpnz_c(:,j+1))'*T213*imag(Ydcpnz_c(:,i+1)));

                    Zdcpnz_c(1,h+1) = Zdcpnz_c(1,h+1) + 0.5*( + real(Xdcpnz_c(:,i+1))'*T321*imag(Ydcpnz_c(:,j+1)) + imag(Xdcpnz_c(:,i+1))'*T321*real(Ydcpnz_c(:,j+1)) ...
                                                              + real(Xdcpnz_c(:,j+1))'*T321*imag(Ydcpnz_c(:,i+1)) + imag(Xdcpnz_c(:,j+1))'*T321*real(Ydcpnz_c(:,i+1)));


                    Zdcpnz_c(1,h+1) = Zdcpnz_c(1,h+1) + 0.5*1i*( - real(Xdcpnz_c(:,i+1))'*T321*real(Ydcpnz_c(:,j+1)) + imag(Xdcpnz_c(:,i+1))'*T321*imag(Ydcpnz_c(:,j+1)) ...
                                                                 - real(Xdcpnz_c(:,j+1))'*T321*real(Ydcpnz_c(:,i+1)) + imag(Xdcpnz_c(:,j+1))'*T321*imag(Ydcpnz_c(:,i+1)));
                    
                    Zdcpnz_c(2,h+1) = Zdcpnz_c(2,h+1) + 0.5*( + real(Xdcpnz_c(:,i+1))'*T132*imag(Ydcpnz_c(:,j+1)) + imag(Xdcpnz_c(:,i+1))'*T132*real(Ydcpnz_c(:,j+1)) ...
                                                              + real(Xdcpnz_c(:,j+1))'*T132*imag(Ydcpnz_c(:,i+1)) + imag(Xdcpnz_c(:,j+1))'*T132*real(Ydcpnz_c(:,i+1)));

                    Zdcpnz_c(2,h+1) = Zdcpnz_c(2,h+1) + 1i*0.5*( - real(Xdcpnz_c(:,i+1))'*T132*real(Ydcpnz_c(:,j+1)) + imag(Xdcpnz_c(:,i+1))'*T132*imag(Ydcpnz_c(:,j+1)) ...
                                                                 - real(Xdcpnz_c(:,j+1))'*T132*real(Ydcpnz_c(:,i+1)) + imag(Xdcpnz_c(:,j+1))'*T132*imag(Ydcpnz_c(:,i+1)));

                end
            end
%%%%%%%%%%%%%%%%%%%%%%%%%%%% h>N  %%%%%%%%%%%%%%%%%%%%%%%%%%%%%%%%%%%%%%%%% 
        else %h>N
            if(HrmDbl)
            
                %%%%%%%%%%%%%%%%%%%%%%%%%%% PP + NN %%%%%%%%%%%%%%%%%%%%%%%%%%%
                for i = h-N : N
                    Zdcpnz_c(1,h+1) = Zdcpnz_c(1,h+1) +    0.5*( real(Xdcpnz_c(2,i+1))*imag(Ydcpnz_c(2,h-i+1)) + imag(Xdcpnz_c(2,i+1))*real(Ydcpnz_c(2,h-i+1)) );
                    Zdcpnz_c(1,h+1) = Zdcpnz_c(1,h+1) + 1i*0.5*( -real(Xdcpnz_c(2,i+1))*real(Ydcpnz_c(2,h-i+1)) + imag(Xdcpnz_c(2,i+1))*imag(Ydcpnz_c(2,h-i+1)) );

                    Zdcpnz_c(2,h+1) = Zdcpnz_c(2,h+1) +    0.5*( real(Xdcpnz_c(1,i+1))*imag(Ydcpnz_c(1,h-i+1)) + imag(Xdcpnz_c(1,i+1))*real(Ydcpnz_c(1,h-i+1)) );
                    Zdcpnz_c(2,h+1) = Zdcpnz_c(2,h+1) + 1i*0.5*( -real(Xdcpnz_c(1,i+1))*real(Ydcpnz_c(1,h-i+1)) + imag(Xdcpnz_c(1,i+1))*imag(Ydcpnz_c(1,h-i+1)) );
                end
                %%%%%%%%%%%%%%%%%%%%%%%%%%% PP + NN %%%%%%%%%%%%%%%%%%%%%%%%%%%

                if(mod(h,2)==1) %%%%%%%%%%% h>N ODD %%%%%%%%%%%%%%%%%%%

                    for k = (h-1)/2:-1:h-N
                        i = k;  %%%
                        j = h-i;

                        Zdcpnz_c(1,h+1) = Zdcpnz_c(1,h+1) + 0.5*( + real(Xdcpnz_c([1,3],i+1))'*imag(Ydcpnz_c([3,1],j+1)) + imag(Xdcpnz_c([1,3],i+1))'*real(Ydcpnz_c([3,1],j+1)) ...
                                                                  + real(Xdcpnz_c([1,3],j+1))'*imag(Ydcpnz_c([3,1],i+1)) + imag(Xdcpnz_c([1,3],j+1))'*real(Ydcpnz_c([3,1],i+1)));

                        Zdcpnz_c(1,h+1) = Zdcpnz_c(1,h+1) + 1i*0.5*( - real(Xdcpnz_c([1,3],i+1))'*real(Ydcpnz_c([3,1],j+1)) + imag(Xdcpnz_c([1,3],i+1))'*imag(Ydcpnz_c([3,1],j+1)) ...
                                                                     - real(Xdcpnz_c([1,3],j+1))'*real(Ydcpnz_c([3,1],i+1)) + imag(Xdcpnz_c([1,3],j+1))'*imag(Ydcpnz_c([3,1],i+1)));

                        Zdcpnz_c(2,h+1) = Zdcpnz_c(2,h+1) + 0.5*( + real(Xdcpnz_c([2,3],i+1))'*imag(Ydcpnz_c([3,2],j+1)) + imag(Xdcpnz_c([2,3],i+1))'*real(Ydcpnz_c([3,2],j+1)) ...
                                                                  + real(Xdcpnz_c([2,3],j+1))'*imag(Ydcpnz_c([3,2],i+1)) + imag(Xdcpnz_c([2,3],j+1))'*real(Ydcpnz_c([3,2],i+1)));

                        Zdcpnz_c(2,h+1) = Zdcpnz_c(2,h+1) + 1i*0.5*( - real(Xdcpnz_c([2,3],i+1))'*real(Ydcpnz_c([3,2],j+1)) + imag(Xdcpnz_c([2,3],i+1))'*imag(Ydcpnz_c([3,2],j+1)) ...
                                                                     - real(Xdcpnz_c([2,3],j+1))'*real(Ydcpnz_c([3,2],i+1)) + imag(Xdcpnz_c([2,3],j+1))'*imag(Ydcpnz_c([3,2],i+1)));

                        Zdcpnz_c(3,h+1) = Zdcpnz_c(3,h+1) +    0.5*(+real(Xdcpnz_c(:,i+1))'*T213*imag(Ydcpnz_c(:,j+1)) + real(Xdcpnz_c(:,j+1))'*T213*imag(Ydcpnz_c(:,i+1)) + imag(Xdcpnz_c(:,i+1))'*T213*real(Ydcpnz_c(:,j+1)) + imag(Xdcpnz_c(:,j+1))'*T213*real(Ydcpnz_c(:,i+1)));
                        Zdcpnz_c(3,h+1) = Zdcpnz_c(3,h+1) + 1i*0.5*(-real(Xdcpnz_c(:,i+1))'*T213*real(Ydcpnz_c(:,j+1)) - real(Xdcpnz_c(:,j+1))'*T213*real(Ydcpnz_c(:,i+1)) + imag(Xdcpnz_c(:,i+1))'*T213*imag(Ydcpnz_c(:,j+1)) + imag(Xdcpnz_c(:,j+1))'*T213*imag(Ydcpnz_c(:,i+1)));

                    end

                else %%%%%%%%%%% h>N EVEN %%%%%%%%%%%%%%%%%%%

                    Zdcpnz_c(1,h+1) = 0.5*real(Xdcpnz_c(:,h/2+1))'*T321*imag(Ydcpnz_c(:,h/2+1)) + 0.5*imag(Xdcpnz_c(:,h/2+1))'*T321*real(Ydcpnz_c(:,h/2+1)) - 0.5*1i*real(Xdcpnz_c(:,h/2+1))'*T321*real(Ydcpnz_c(:,h/2+1)) + 0.5*1i*imag(Xdcpnz_c(:,h/2+1))'*T321*imag(Ydcpnz_c(:,h/2+1));
                    Zdcpnz_c(2,h+1) = 0.5*real(Xdcpnz_c(:,h/2+1))'*T132*imag(Ydcpnz_c(:,h/2+1)) + 0.5*imag(Xdcpnz_c(:,h/2+1))'*T132*real(Ydcpnz_c(:,h/2+1))- 0.5*1i*real(Xdcpnz_c(:,h/2+1))'*T132*real(Ydcpnz_c(:,h/2+1)) + 0.5*1i*imag(Xdcpnz_c(:,h/2+1))'*T132*imag(Ydcpnz_c(:,h/2+1));
                    Zdcpnz_c(3,h+1) = Zdcpnz_c(3,h+1) + 0.5*imag(Xdcpnz_c(3,h/2+1)*Ydcpnz_c(3,h/2+1)) - 1i*0.5*real(Xdcpnz_c(3,h/2+1)*Ydcpnz_c(3,h/2+1));


                    for i = (h+2)/2:N
                        j = h-i;

                        Zdcpnz_c(1,h+1) = Zdcpnz_c(1,h+1) + 0.5*( + real(Xdcpnz_c(:,i+1))'*T321*imag(Ydcpnz_c(:,j+1)) + imag(Xdcpnz_c(:,i+1))'*T321*real(Ydcpnz_c(:,j+1)) ...
                                                                  + real(Xdcpnz_c(:,j+1))'*T321*imag(Ydcpnz_c(:,i+1)) + imag(Xdcpnz_c(:,j+1))'*T321*real(Ydcpnz_c(:,i+1)));
    
                        Zdcpnz_c(1,h+1) = Zdcpnz_c(1,h+1) + 0.5*1i*( - real(Xdcpnz_c(:,i+1))'*T321*real(Ydcpnz_c(:,j+1)) + imag(Xdcpnz_c(:,i+1))'*T321*imag(Ydcpnz_c(:,j+1)) ...
                                                                     - real(Xdcpnz_c(:,j+1))'*T321*real(Ydcpnz_c(:,i+1)) + imag(Xdcpnz_c(:,j+1))'*T321*imag(Ydcpnz_c(:,i+1)));

                        Zdcpnz_c(2,h+1) = Zdcpnz_c(2,h+1) + 0.5*( + real(Xdcpnz_c(:,i+1))'*T132*imag(Ydcpnz_c(:,j+1)) + imag(Xdcpnz_c(:,i+1))'*T132*real(Ydcpnz_c(:,j+1)) ...
                                                                  + real(Xdcpnz_c(:,j+1))'*T132*imag(Ydcpnz_c(:,i+1)) + imag(Xdcpnz_c(:,j+1))'*T132*real(Ydcpnz_c(:,i+1)));
    
                        Zdcpnz_c(2,h+1) = Zdcpnz_c(2,h+1) + 0.5*1i*( - real(Xdcpnz_c(:,i+1))'*T132*real(Ydcpnz_c(:,j+1)) + imag(Xdcpnz_c(:,i+1))'*T132*imag(Ydcpnz_c(:,j+1)) ...
                                                                     - real(Xdcpnz_c(:,j+1))'*T132*real(Ydcpnz_c(:,i+1)) + imag(Xdcpnz_c(:,j+1))'*T132*imag(Ydcpnz_c(:,i+1)));

                        Zdcpnz_c(3,h+1) = Zdcpnz_c(3,h+1) +    0.5*(+real(Xdcpnz_c(:,i+1))'*T213*imag(Ydcpnz_c(:,j+1)) + real(Xdcpnz_c(:,j+1))'*T213*imag(Ydcpnz_c(:,i+1)) + imag(Xdcpnz_c(:,i+1))'*T213*real(Ydcpnz_c(:,j+1)) + imag(Xdcpnz_c(:,j+1))'*T213*real(Ydcpnz_c(:,i+1)));
                        Zdcpnz_c(3,h+1) = Zdcpnz_c(3,h+1) + 1i*0.5*(-real(Xdcpnz_c(:,i+1))'*T213*real(Ydcpnz_c(:,j+1)) - real(Xdcpnz_c(:,j+1))'*T213*real(Ydcpnz_c(:,i+1)) + imag(Xdcpnz_c(:,i+1))'*T213*imag(Ydcpnz_c(:,j+1)) + imag(Xdcpnz_c(:,j+1))'*T213*imag(Ydcpnz_c(:,i+1)));

                    end
                end
            end
        end  
    end
    

end

== matlab function DQN_Lib/DQn->ABC6 ==
  data: Xdcpnz_c input; tho input; Xabc output; N parameter
%function abc = Mult(Z0,Zdp,Zqp,Zdn,Zqn,Zdz,Zqz,th, N)
function Xabc = dqn2abc(Xdcpnz_c,tho,N)

    persistent Sas;
    persistent Ssa;

    if(isempty(Sas)) 
        a = -0.5+0.866i;
        a2 = -0.5-0.866i;
        Sas = [1,a,a2;1,a2,a;1,1,1]/3;
        Ssa = eye(3)/(Sas);
    end

    Xabc = zeros(3,1);

    for i = 1 : N+1
    
    
        if(i>1)
            h = i-1;
    
            th = h*tho;
        
            mag_p = abs(Xdcpnz_c(1,i));
            ang_p = angle(Xdcpnz_c(1,i));
            mag_n = abs(Xdcpnz_c(2,i));
            ang_n = angle(Xdcpnz_c(2,i));
            mag_z = abs(Xdcpnz_c(3,i));
            ang_z = angle(Xdcpnz_c(3,i));
            
            abc3p = mag_p*[sin(th+ang_p) ; sin(th+ang_p-2*pi/3) ; sin(th+ang_p+2*pi/3) ];
            abc3n = mag_n*[sin(th+ang_n) ; sin(th+ang_n+2*pi/3) ; sin(th+ang_n-2*pi/3) ];
            abc3z = mag_z*[sin(th+ang_z) ; sin(th+ang_z)        ; sin(th+ang_z)  ];
        
            Xabc = Xabc + abc3p+abc3n+abc3z;
        else
            Xabc = Xabc + real(Ssa*(Xdcpnz_c(:,1)));
        
        end
    
        
    end

end

== matlab function DQN_Lib/Der_DQNc_Mat ==
  data: Xpnz input; N parameter; Zpnz output; w parameter; EMT parameter; Ts parameter; sw_soft parameter
function Zpnz    = fMultDQNc(Xpnz, N, w, EMT, Ts, sw_soft)
    Zpnz = complex(zeros(3,N+1));

    sX = size(Xpnz,2);
    Xpnz = [Xpnz zeros(3,N+1-sX)];

    persistent Xpnz_old;
    persistent firstStep;

    if(isempty(Xpnz_old)) 
        Xpnz_old = complex(zeros(3,N+1));
        firstStep = 0;

    end


        for h = 2 : N + 1
            wn = (h-1)*w;
            if(EMT)
                if(sw_soft==1 && firstStep == 0)
                    Xpnz_old(:,h) = Xpnz(:,h);
                else
                    Zpnz(:,h) = (Xpnz(:,h)-Xpnz_old(:,h))/Ts;
                    Xpnz_old(:,h) = Xpnz(:,h);
                end

            end

            Zpnz(:,h) = Zpnz(:,h) + 1i*wn*Xpnz(:,h);

            firstStep = 1;
        end
    
end

== matlab function DQN_Lib/Gain_DQNc_Mat ==
  data: Xpnz input; Ypnz output; Rabc parameter; chkInv parameter; HRM parameter
function Ypnz  = Gain_Mat2(Xpnz, Rabc, chkInv, HRM)
    persistent Rpnz;
    %persistent nrInp;
    persistent nrOut;

    mrows = size(Rabc,1)/3; %signal size
    mcols = size(Rabc,2)/3; %signal size

    nrInp = size(Rabc,1);

    % Ypnz = complex(zeros(nrInp, HRM+1));


    if(isempty(Rpnz)) 

        Rpnz = complex(zeros(3*mrows,3*mcols));
        a = -0.5+0.866i;
        a2 = -0.5-0.866i;
        Sas = [1,a,a2;1,a2,a;1,1,1]/3;
        %Ssa = eye(3)/(Sas);
        %nrInp = size(Xpnz,1) / 3;

        for i = 1 : mrows
            for j = 1 : mcols
                Rpnz((1:3) + (i-1)*3,(1:3) + (j-1)*3) = Sas*Rabc((1:3) + (i-1)*3,(1:3) + (j-1)*3)/Sas;
            end
        end

        if(chkInv)
            %Rpnz((1:3) + (i-1)*3,(1:3) + (j-1)*3) = eye(3)/Rpnz((1:3) + (i-1)*3,(1:3) + (j-1)*3);
            Rpnz = eye(3*mrows,3*mcols)/Rpnz;
        end

    end




    
    Ypnz = Rpnz*Xpnz;

end

== matlab function DQN_Lib/Int_DQNc_Mat ==
  settings: updateMethod=DISCRETE
  data: Xpnz input; N parameter; dt parameter; w parameter; InitInt parameter; Zpnz output; R parameter; iL parameter; swFeed parameter
function Zpnz    = Int_DQN_Mat(Xpnz, N, dt, w, InitInt, R, iL, swFeed)


    nrSig = size(Xpnz,1)/3;
    Zpnz = complex(zeros(nrSig*3,N+1));

    persistent Zpnz_old;
    persistent Xpnz_old;
    persistent Krl1;
    persistent Krl2;
    persistent dt2;
        
    if(isempty(Zpnz_old)) 
    


        
        % if(~isempty(InitInt))
        % Zpnz_old(:,1) = Sas * InitInt;
        % end


        Zpnz_old = complex(zeros(nrSig*3,N+1));
        Xpnz_old = complex(zeros(nrSig*3,N+1));
        dt2 = dt/2;

        if(swFeed)
            mrows = size(R,1)/3; %signal size
            mcols = size(R,2)/3; %signal size

            szMatR = size(R,1);
            szMatiL = size(iL,1);

            if(szMatiL ~= szMatR || size(R,1) ~= size(R,2) || size(iL,1) ~= size(iL,2))
                error('[Int_DQN_Mat/swFeedback] check matrix sizes!');
            end
    
            Rpnz = complex(zeros(3*mrows,3*mcols));
            iLpnz = complex(zeros(3*mrows,3*mcols));

            a = -0.5+0.866i;
            a2 = -0.5-0.866i;
            Sas = [1,a,a2;1,a2,a;1,1,1]/3;
    
            for i = 1 : mrows
                for j = 1 : mcols
                     Rpnz((1:3) + (i-1)*3,(1:3) + (j-1)*3) = Sas*R((1:3) + (i-1)*3,(1:3) + (j-1)*3)/Sas;
                    iLpnz((1:3) + (i-1)*3,(1:3) + (j-1)*3) = Sas*iL((1:3) + (i-1)*3,(1:3) + (j-1)*3)/Sas;
                end
            end

            Rpnz  = diag(diag(real(Rpnz)));
            iLpnz = diag(diag(real(iLpnz)));

            Krl1 = (iLpnz/(eye(szMatR)+dt2*Rpnz*iLpnz));
            Krl2 = (eye(szMatR)-dt2*Rpnz*iLpnz)/(eye(szMatR)+dt2*Rpnz*iLpnz);
        else
            Krl1 = 1;
            Krl2 = 1;
        end
            
    end

    if(swFeed)
        Zpnz(:,1) = Krl1*dt2*(Xpnz(:,1)+Xpnz_old(:,1))+Krl2*Zpnz_old(:,1);
    else
        Zpnz(:,1) = dt2*(Xpnz(:,1)+Xpnz_old(:,1))+Zpnz_old(:,1);
    end

    Xpnz_old(:,1) = Xpnz(:,1);
    Zpnz_old(:,1) = Zpnz(:,1);

    for i = 1 : N
        if(N>0)
            wn =  i * w; 
            wndt2 = wn*dt2;

            A = 2*dt2/(1+wndt2^2);
            B = (1-wndt2^2)/(1+wndt2^2);

            if(swFeed)

                Zpnz(:,i+1) =      Krl1*A*(real(Xpnz(:,i+1))+wndt2*imag(Xpnz(:,i+1)))+Krl2*(B*real(Zpnz_old(:,i+1))+A*wn*imag(Zpnz_old(:,i+1))) ...
                             + 1i*(Krl1*A*(imag(Xpnz(:,i+1))-wndt2*real(Xpnz(:,i+1)))+Krl2*(B*imag(Zpnz_old(:,i+1))-A*wn*real(Zpnz_old(:,i+1))));
            else
                Zpnz(:,i+1) =      A*(real(Xpnz(:,i+1))+wndt2*imag(Xpnz(:,i+1)))+(B*real(Zpnz_old(:,i+1))+A*wn*imag(Zpnz_old(:,i+1))) ...
                             + 1i*(A*(imag(Xpnz(:,i+1))-wndt2*real(Xpnz(:,i+1)))+(B*imag(Zpnz_old(:,i+1))-A*wn*real(Zpnz_old(:,i+1))));
            end

            Zpnz_old(:,i+1) = Zpnz(:,i+1);

        end
    end


end

== matlab function DQN_Lib/SS_DQNc_Mat ==
  settings: updateMethod=DISCRETE
  data: Xpnz input; N parameter; dt parameter; w parameter; x0 parameter; Zopnz output; A parameter; B parameter; C parameter; D parameter
function Zopnz    = Int_DQN_Mat(Xpnz, N, dt, w, x0, A, B, C, D)


    persistent Zpnz_old;
    persistent Xpnz_old;
    persistent Krl1;
    persistent Krl2;
    persistent dt2;
    persistent Bpnz;
    persistent Cpnz;
    persistent Dpnz;
        
%%%%%%%%%%%%%%%%%%%%%%%%%%%%%%%%%%%%%%%%%%%%%% INITIAL CONDITIONS %%%%%%%%%%%%%%%%%%%%%%%%%%%%%%%%%%%%%%%%%%%%%%

    if(isempty(Zpnz_old)) 
    


        dt2 = dt/2;

        a = -0.5+0.866i;
        a2 = -0.5-0.866i;
        Sas = [1,a,a2;1,a2,a;1,1,1]/3;

        arows = size(A,1)/3; %signal size
        acols = size(A,2)/3; %signal size

        brows = size(B,1)/3; %signal size
        bcols = size(B,2)/3; %signal size

        crows = size(C,1)/3; %signal size
        ccols = size(C,2)/3; %signal size

        drows = size(D,1)/3; %signal size
        dcols = size(D,2)/3; %signal size

        Apnz = complex(zeros(3*arows,3*acols));

        Zpnz_old = complex(zeros(brows*3,N+1));
        Xpnz_old = complex(zeros(brows*3,N+1));


        %%%%%%%%%%%%%%%%%%%%%%% Check for inconsistencies  %%%%%%%%%%%%%%%%%%%%%%%

        szMatA = size(A,1);
        iL = eye(szMatA);
        szMatiL = size(iL,1);

        if(szMatiL ~= szMatA || size(A,1) ~= size(A,2) || size(iL,1) ~= size(iL,2))
            error('[Int_DQN_Mat/swFeedback] check matrix A size!');
        end

        if(arows ~= brows || acols ~= ccols || crows ~= drows || bcols ~= dcols)
            error('[Int_DQN_Mat/Initialize] the sizes of the state-space matrices!');
        end

        %%%%%%%%%%%%%%%%%%%%%%%%%%%%%%%%%%%%%%%%%%%%%%%%%%%%%%%%%%%%%%%

        %%%%%%%%%%%%%%%%%%%%%%% A --> Bpnz %%%%%%%%%%%%%%%%%%%%%%%
        for i = 1 : arows
            for j = 1 : acols
                Apnz((1:3) + (i-1)*3,(1:3) + (j-1)*3) = -Sas*A((1:3) + (i-1)*3,(1:3) + (j-1)*3)/Sas; %Negative A (-A)
                Apnz((1:3) + (i-1)*3,(1:3) + (j-1)*3) = diag(diag(real(Apnz((1:3) + (i-1)*3,(1:3) + (j-1)*3))));
            end
        end

        Apnz = real(Apnz);

        Krl1 = (iL+dt2*Apnz);
        Krl2 = (iL-dt2*Apnz)/(iL+dt2*Apnz);
        %%%%%%%%%%%%%%%%%%%%%%%%%%%%%%%%%%%%%%%%%%%%%%%%%%%%%%%%%%%%%%%

        %%%%%%%%%%%%%%%%%%%%%%% B --> Bpnz %%%%%%%%%%%%%%%%%%%%%%%

        Bpnz = complex(zeros(3*brows,3*bcols));

        for i = 1 : brows
            for j = 1 : bcols
                Bpnz((1:3) + (i-1)*3,(1:3) + (j-1)*3) = Sas*B((1:3) + (i-1)*3,(1:3) + (j-1)*3)/Sas;
            end
        end
        %%%%%%%%%%%%%%%%%%%%%%%%%%%%%%%%%%%%%%%%%%%%%%%%%%%%%%%%%%%%%%%

        %%%%%%%%%%%%%%%%%%%%%%% C --> Cpnz %%%%%%%%%%%%%%%%%%%%%%%

        Cpnz = complex(zeros(3*crows,3*ccols));

        for i = 1 : crows
            for j = 1 : ccols
                Cpnz((1:3) + (i-1)*3,(1:3) + (j-1)*3) = Sas*C((1:3) + (i-1)*3,(1:3) + (j-1)*3)/Sas;
            end
        end
        %%%%%%%%%%%%%%%%%%%%%%%%%%%%%%%%%%%%%%%%%%%%%%%%%%%%%%%%%%%%%%%

        %%%%%%%%%%%%%%%%%%%%%%% C --> Cpnz %%%%%%%%%%%%%%%%%%%%%%%

        Dpnz = complex(zeros(3*drows,3*dcols));

        for i = 1 : drows
            for j = 1 : dcols
                Dpnz((1:3) + (i-1)*3,(1:3) + (j-1)*3) = Sas*D((1:3) + (i-1)*3,(1:3) + (j-1)*3)/Sas;
            end
        end
        %%%%%%%%%%%%%%%%%%%%%%%%%%%%%%%%%%%%%%%%%%%%%%%%%%%%%%%%%%%%%%%


        %%%%%%%%%%%%%%%%%%%%%%% x0 --> Zpnz_old %%%%%%%%%%%%%%%%%%%%%%%
        if(~isempty(x0))
            % Zpnz_old = x0;

            x0 = x0;
            if(mod(numel(x0),3)~=0) error('[SS_DQNc_Mat] x0 vector with wrong size --> needs to be a multiple of 3!'); end
    
            for k = 1 : numel(x0)/3
                % mag_p = abs(sum(x0((k-1)*3+1:(k-1)*3+3)'.*exp(1i*[0 -2*pi/3 2*pi/3]))'*(2/3));
                % th = asin(real(x0((k-1)*3+1)/(mag_p)));
                % Zpnz_old((k-1)*3+1,1) = imag(mag_p*exp(1i*th));
                % Zpnz_old((k-1)*3+1:(k-1)*3+3,1) = ([2.0995 + 0.4189i;2.0995 - 0.4189i;0]*1e3);
                Zpnz_old((k-1)*3+1:(k-1)*3+3,1) = Sas*x0((k-1)*3+1:(k-1)*3+3);
            end
        end
        %%%%%%%%%%%%%%%%%%%%%%%%%%%%%%%%%%%%%%%%%%%%%%%%%%%%%%%%%%%%%%%
           
    end

%%%%%%%%%%%%%%%%%%%%%%%%%%%%%%%%%%%%%%%%%%%%%%%%%%%%%%%%%%%%%%%%%%%%%%%%%%%%%%%%%%%%%%%%%%%%%%%%%%%%%%%%%%%%%%%%%%%

    nrIn = size(B,1)/3;
    nrOut = size(C,1)/3;

    % Zopnz = complex(zeros(nrOut*3,N+1));
    % Xbpnz = complex(zeros(nrIn*3,N+1));

    Zipnz = complex(zeros(nrIn*3,N+1));

    Xbpnz = Bpnz*Xpnz; %Multiply with the B matrix


    %%%%%%%%%%%%%%%%%%%%%%% Integration with feedback loop %%%%%%%%%%%%%%%%%%%%%%%
    Zipnz(:,1) = Krl1*dt2*(Xbpnz(:,1)+Xpnz_old(:,1))+Krl2*Zpnz_old(:,1);

    Xpnz_old(:,1) = Xbpnz(:,1);
    Zpnz_old(:,1) = Zipnz(:,1);

    for i = 1 : N
        if(N>0)
            wn      =  i * w; 
            wndt2   = wn*dt2;

            Ai      = 2*dt2/(1+wndt2^2);
            Bi      = (1-wndt2^2)/(1+wndt2^2);

            Zipnz(:,i+1) =      Krl1*Ai*(real(Xbpnz(:,i+1))+wndt2*imag(Xbpnz(:,i+1)))+Krl2*(Bi*real(Zpnz_old(:,i+1))+Ai*wn*imag(Zpnz_old(:,i+1))) ...
                         + 1i*(Krl1*Ai*(imag(Xbpnz(:,i+1))-wndt2*real(Xbpnz(:,i+1)))+Krl2*(Bi*imag(Zpnz_old(:,i+1))-Ai*wn*real(Zpnz_old(:,i+1))));

            Zpnz_old(:,i+1) = Zipnz(:,i+1);
        end
    end

    %%%%%%%%%%%%%%%%%%%%%%%%%%%%%%%%%%%%%%%%%%%%%%%%%%%%%%%%%%%%%%%

    %
    %Zopnz = -Cpnz*Zipnz;

    if(any(D,'all'))
        Zopnz = -Cpnz*Zipnz + Dpnz*Xpnz; %Multiply with the C matrix
    else
        Zopnz = -Cpnz*Zipnz;
    end

end
